simulink model "Copy_2_of_continuos_plant"  (R2016b)
settings: Solver=ode15s  StartTime=0.0  StopTime=200  FixedStep=0.01  RelTol=10^-1  AbsTol=10^-1
undefined symbols (not defined in the file or in its folder): deg, rad, s
libraries: simulink x6, aerolibconvert2 x2, dspsrcs4 x1, aerolib6dof2 x1
settings Model: Creator=Utente  LastModifiedBy=liana
settings SolverCC: SolverJacobianMethodControl=SparsePerturbation  SolverResetMethod=Robust
settings DataIOCC: SaveState=on
settings OptimizationCC: BlockReduction=off  DefaultParameterBehavior=Inlined  BufferReuse=off

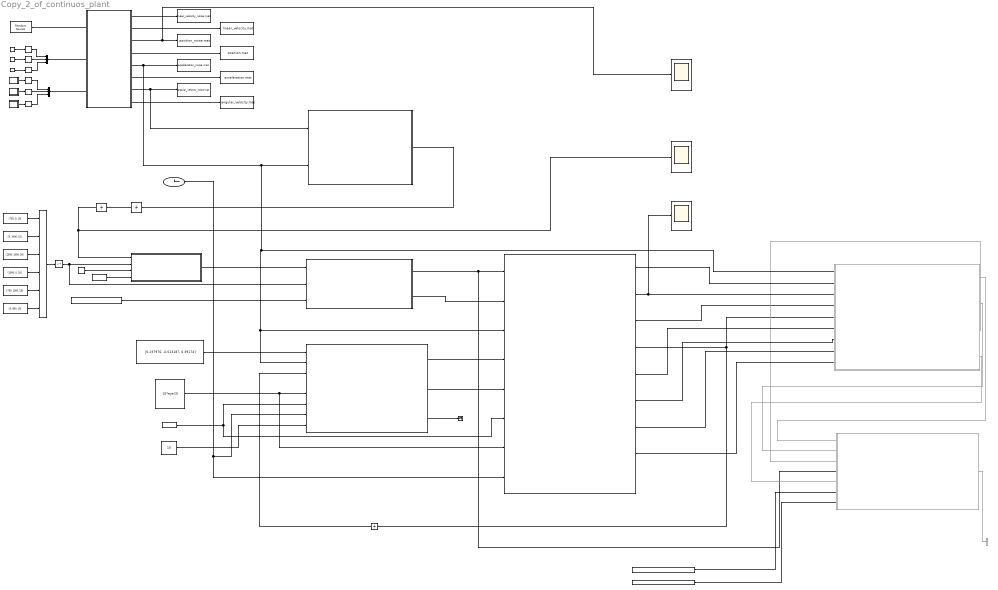
== system Copy_2_of_continuos_plant ==
  Attitude Observer : Subsystem
  Clock : Clock
      settings: Decimation=50
  Const : Constant
  Const1 : Constant  Value=0
  Const2 : Constant  Value=0
  Fx Slider : simulink/Math Operations/Slider Gain  low=-1  gain=1  high=1
  Fy Slider : simulink/Math Operations/Slider Gain  low=-1  gain=0  high=1
  Fz Slider : simulink/Math Operations/Slider Gain  low=-1  gain=0  high=1
  Integrator1 : Integrator  AbsoluteTolerance=10^-3
  Integrator2 : Integrator  AbsoluteTolerance=10^-3
  Kalman - Bucy Filter : Subsystem  Commented=on
  Kp : Constant  Value=10*eye(3)
  Local linearization1 : Subsystem  Commented=on
  Math Function : Math  Operator=transpose  SaturateOnIntegerOverflow=on
  Matrix Concatenate (transponders positions) : Concatenate  NumInputs=6  Mode=Multidimensional array  ConcatenateDimension=2
  Mechanisation subsystem : Subsystem
  Mux : Mux  Inputs=3
  Mux1 : Mux  Inputs=3
  Mxx Slider : simulink/Math Operations/Slider Gain  low=0  gain=0  high=1
  Myy Slider : simulink/Math Operations/Slider Gain  low=0  gain=0  high=1
  Mzz Slider : simulink/Math Operations/Slider Gain  low=-1  gain=1  high=3
  Nonlinear algebraic transform and solution : Subsystem
  Pitch moment : Subsystem  mask(timed input){t=[0 3 3 4 4 5 5  7.5 7.5 8.5 8.5 9.5 9.5 10], u=[0 0  1 1 -1 -1.005 0 0 -1 -1 1 1 0 0]*3.138/2}
      mask prompts: t "time values:"; u "input values"
      mask Display: plot(t,u)
  Position TMO : Scope
  "Position mechanisation " : Scope
  Position trajectory : Scope
  Q matrix : Constant  Value=diag([0, 0, 0, 10^-5, 10^-3, 10^-3, 10^-3, 10^-8, 10^-8, 10^-8])
  R matrix : Constant  Value=0.25*diag([1 1 1 1])
  Random Source : dspsrcs4/Random Source  SrcType=Gaussian  NormMethod=Ziggurat  CltLength=12  MinVal=0  MaxVal=1  MeanVal=[0.05 0.05 0.05]  VarVal=[5 5 5]  RepMode=Not repeatable  rawSeed=1  IsInherit=off  SampMode=Discrete  SampTime=1  SampFrame=1  DataType=Double  OutComplex=Real  OutputFrames=off
  Roll moment : Subsystem  mask(timed input){t=[0 1 1 2 2  10], u=[1 1 -1 -.998  0 0]*3.144/2}
      mask prompts: t "time values:"; u "input values"
      mask Display: plot(t,u)
  Terminator : Terminator
  Terminator2 : Terminator  Commented=on
  Translational Motion Observer : Subsystem
  Unit Delay : UnitDelay  SampleTime=-1
  Yaw moment : Subsystem  mask(timed input){t=[0 6 6 7 7 8 8 10], u=[0 0  -1 -1 1 1 0 0]*3.1/2}
      mask prompts: t "time values:"; u "input values"
      mask Display: plot(t,u)
  acceleration file : ToFile  Filename=acceleration_noise.mat  MatrixName=acc  SaveFormat=Timeseries
  acceleration file2 : ToFile  Filename=acceleration.mat  MatrixName=acc  SaveFormat=Timeseries
  angular velocity file : ToFile  Filename=angular_velocity_noise.mat  MatrixName=av  SaveFormat=Timeseries
  angular velocity file1 : ToFile  Filename=angular_velocity.mat  MatrixName=av  SaveFormat=Timeseries
  beta : Constant  Value=100
  epsilon : Constant  Value=[1 1 1 1 1 1]*0.1
  ki : Constant  Value=10
  magneto_values (Pisa) : Constant  Value=[0.237976, -0.013187, 0.39174]'
  p_n_1 : Constant  Value=[750, 0, 10]
  p_n_2 : Constant  Value=[0, 1000, 15]
  p_n_3 : Constant  Value=[1500, 1000, 30]
  p_n_4 : Constant  Value=[1500, 0, 20]
  p_n_5 : Constant  Value=[750, 1000, 25]
  p_n_6 : Constant  Value=[0, 600, 10]
  position file : ToFile  Filename=position_noise.mat  MatrixName=pos_noise  SaveFormat=Timeseries
  position file1 : ToFile  Filename=position.mat  MatrixName=pos  SaveFormat=Timeseries
  position_0_fixed_reference : Constant  Value=[4 5 5]
  pseudorange_measurement_model : MATLAB Function  TreatAsAtomicUnit=on
  sigma : Constant  Value=0.25
  trajectory : Subsystem
  velocity file : ToFile  Filename=linear_velocity_noise.mat  MatrixName=lv  SaveFormat=Timeseries
  velocity file1 : ToFile  Filename=linear_velocity.mat  MatrixName=lv  SaveFormat=Timeseries
  wires:
  Clock/1 -> Translational Motion Observer/8(t), Attitude Observer/7(t)
  Mechanisation subsystem/1(v_n_dot) -> Integrator1/1
  Nonlinear algebraic transform and solution/1(delta) -> Kalman - Bucy Filter/4(sensors measurements), Translational Motion Observer/1(delta)
  Translational Motion Observer/4(f_n_stim) -> Local linearization1/5(f_n_stim), Unit Delay/1
  Attitude Observer/1(J) -> Translational Motion Observer/4(J)
  Attitude Observer/2(R_nb_stim) -> Translational Motion Observer/5(R_nb_stim)
  Attitude Observer/3(b_stim) -> Terminator/1
  Kp/1 -> Translational Motion Observer/7(Kp), Attitude Observer/5(Kp)
  sigma/1 -> Attitude Observer/6(sigma), Translational Motion Observer/6(sigma)
  Translational Motion Observer/3(v_n_stim) -> Local linearization1/4(v_n_stim)
  Nonlinear algebraic transform and solution/2(C_dx) -> Translational Motion Observer/2(C_dx)
  Local linearization1/1(AL) -> Kalman - Bucy Filter/1(AL)
  Local linearization1/2(BL) -> Kalman - Bucy Filter/2(BL)
  Local linearization1/3(CL) -> Kalman - Bucy Filter/3(CL)
  pseudorange_measurement_model/1(y) -> Nonlinear algebraic transform and solution/1(y)
  Local linearization1/4(U) -> Kalman - Bucy Filter/5(U)
  beta/1 -> pseudorange_measurement_model/3(beta)
  epsilon/1 -> pseudorange_measurement_model/4(epsilon)
  Matrix Concatenate (transponders positions)/1 -> Math Function/1
  R matrix/1 -> Kalman - Bucy Filter/6(R)
  Q matrix/1 -> Kalman - Bucy Filter/7(Q)
  Kalman - Bucy Filter/1(Out1) -> Terminator2/1
  Translational Motion Observer/5(K) -> Local linearization1/6(K)
  Translational Motion Observer/6("C ") -> Local linearization1/7(C)
  Translational Motion Observer/7(" A") -> Local linearization1/8(A)
  Translational Motion Observer/8(B) -> Local linearization1/9(B)
  ki/1 -> Attitude Observer/8(Ki)
  Unit Delay/1 -> Attitude Observer/3(f_n_stim)
  Translational Motion Observer/1(beta_stim) -> Local linearization1/2(beta_stim)
  Translational Motion Observer/2(p_n_delta_stim) -> Position TMO/1, Local linearization1/3(p_n_stim)
  p_n_5/1 -> Matrix Concatenate (transponders positions)/5
  p_n_4/1 -> Matrix Concatenate (transponders positions)/4
  p_n_3/1 -> Matrix Concatenate (transponders positions)/3
  p_n_2/1 -> Matrix Concatenate (transponders positions)/2
  p_n_1/1 -> Matrix Concatenate (transponders positions)/1
  Math Function/1 -> pseudorange_measurement_model/2(p_n_i), Nonlinear algebraic transform and solution/2(p)
  trajectory/5(Acceleration_noise) -> Attitude Observer/2(f_b), Translational Motion Observer/3(f_b_imu), Local linearization1/1(f_b_imu), Mechanisation subsystem/2(f_b), acceleration file/1
  position_0_fixed_reference/1 -> Nonlinear algebraic transform and solution/3(p0)
  magneto_values (Pisa)/1 -> Attitude Observer/1(m_b_mag)
  Integrator1/1 -> Integrator2/1
  p_n_6/1 -> Matrix Concatenate (transponders positions)/6
  Integrator2/1 -> pseudorange_measurement_model/1(p_n), "Position mechanisation "/1
  Yaw moment/1(Out1) -> Mzz Slider/1
  Pitch moment/1(Out1) -> Myy Slider/1
  Roll moment/1(Out1) -> Mxx Slider/1
  Const2/1 -> Fz Slider/1
  Const1/1 -> Fy Slider/1
  Const/1 -> Fx Slider/1
  Mzz Slider/1 -> Mux1/3
  Myy Slider/1 -> Mux1/2
  Mxx Slider/1 -> Mux1/1
  Fy Slider/1 -> Mux/2
  Fz Slider/1 -> Mux/3
  Fx Slider/1 -> Mux/1
  Random Source/1 -> trajectory/1(Noise_output)
  Mux/1 -> trajectory/2(Force_xyz)
  Mux1/1 -> trajectory/3(M_xyz)
  trajectory/1(velocity_noise) -> velocity file/1
  trajectory/2(velocity) -> velocity file1/1
  trajectory/4(Position) -> position file1/1
  trajectory/6(Acceleration) -> acceleration file2/1
  trajectory/7(angular_velocity_noise) -> Mechanisation subsystem/1(w_ib), angular velocity file/1
  trajectory/8(angular_velocity) -> angular velocity file1/1
  trajectory/3(Position_noise) -> Position trajectory/1, position file/1

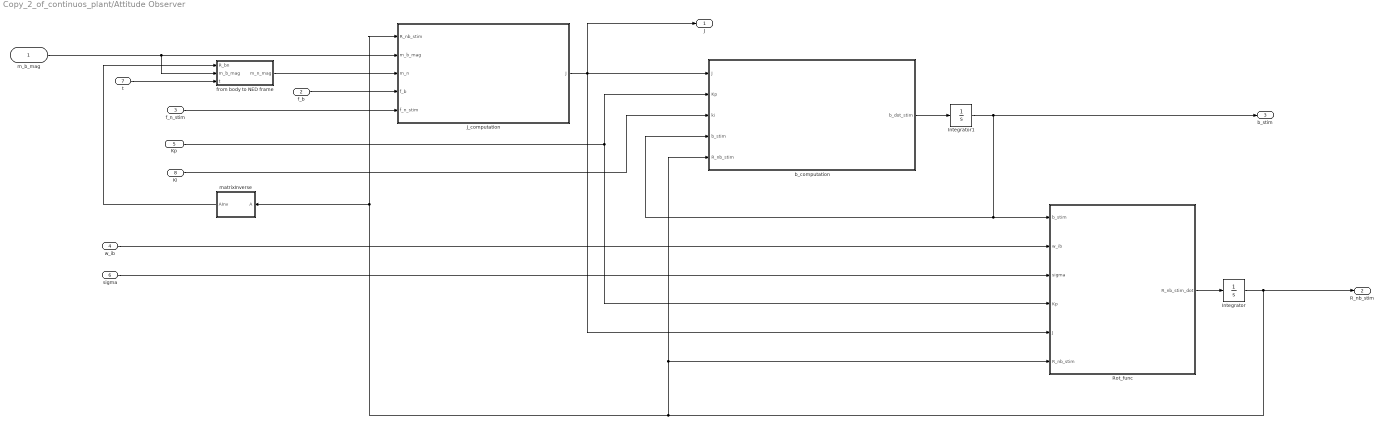
== system Copy_2_of_continuos_plant/Attitude Observer ==
  m_b_mag : Inport
  f_b : Inport  Port=2
  f_n_stim : Inport  Port=3
  w_ib : Inport  Port=4
  Kp : Inport  Port=5
  sigma : Inport  Port=6
  t : Inport  Port=7
  Ki : Inport  Port=8
  Integrator : Integrator  UpperSaturationLimit=1  LowerSaturationLimit=-1  AbsoluteTolerance=10^-1
  Integrator1 : Integrator  UpperSaturationLimit=100  LowerSaturationLimit=-100  AbsoluteTolerance=10^-2
  J_computation : Subsystem
  Rot_func : MATLAB Function  TreatAsAtomicUnit=on
  b_computation : MATLAB Function  TreatAsAtomicUnit=on
  from body to NED frame : MATLAB Function  TreatAsAtomicUnit=on
  matrixInverse : MATLAB Function  TreatAsAtomicUnit=on
  J : Outport
  R_nb_stim : Outport  Port=2
  b_stim : Outport  Port=3
  wires:
  m_b_mag/1 -> from body to NED frame/2(m_b_mag), J_computation/2(m_b_mag)
  from body to NED frame/1(m_n_mag) -> J_computation/3(m_n)
  f_b/1 -> J_computation/4(f_b)
  J_computation/1(J) -> J/1, Rot_func/5(J), b_computation/1(J)
  Kp/1 -> Rot_func/4(Kp), b_computation/2(Kp)
  Ki/1 -> b_computation/3(ki)
  sigma/1 -> Rot_func/3(sigma)
  w_ib/1 -> Rot_func/2(w_ib)
  t/1 -> from body to NED frame/3(t)
  Integrator1/1 -> Rot_func/1(b_stim), b_computation/4(b_stim), b_stim/1
  Integrator/1 -> Rot_func/6(R_nb_stim), b_computation/5(R_nb_stim), matrixInverse/1(A), J_computation/1(R_nb_stim), R_nb_stim/1
  b_computation/1(b_dot_stim) -> Integrator1/1
  Rot_func/1(R_nb_stim_dot) -> Integrator/1
  matrixInverse/1(AInv) -> from body to NED frame/1(R_bn)
  f_n_stim/1 -> J_computation/5(f_n_stim)

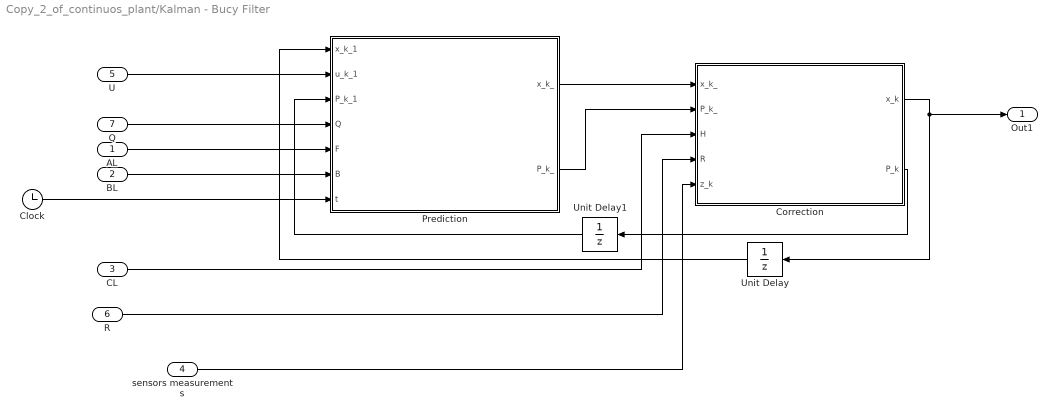
== system Copy_2_of_continuos_plant/Kalman - Bucy Filter ==
  AL : Inport
  BL : Inport  Port=2
  CL : Inport  Port=3
  sensors measurements : Inport  Port=4
  U : Inport  Port=5
  R : Inport  Port=6
  Q : Inport  Port=7
  Clock : Clock
  Correction : MATLAB Function  TreatAsAtomicUnit=on
  Prediction : MATLAB Function  TreatAsAtomicUnit=on
  Unit Delay : UnitDelay  SampleTime=-1
  Unit Delay1 : UnitDelay  SampleTime=-1
  Out1 : Outport
  wires:
  Prediction/2(P_k_) -> Correction/2(P_k_)
  Prediction/1(x_k_) -> Correction/1(x_k_)
  Correction/2(P_k) -> Unit Delay1/1
  Correction/1(x_k) -> Unit Delay/1, Out1/1
  AL/1 -> Prediction/5(F)
  CL/1 -> Correction/3(H)
  Clock/1 -> Prediction/7(t)
  Q/1 -> Prediction/4(Q)
  sensors measurements/1 -> Correction/5(z_k)
  BL/1 -> Prediction/6(B)
  U/1 -> Prediction/2(u_k_1)
  R/1 -> Correction/4(R)
  Unit Delay/1 -> Prediction/1(x_k_1)
  Unit Delay1/1 -> Prediction/3(P_k_1)

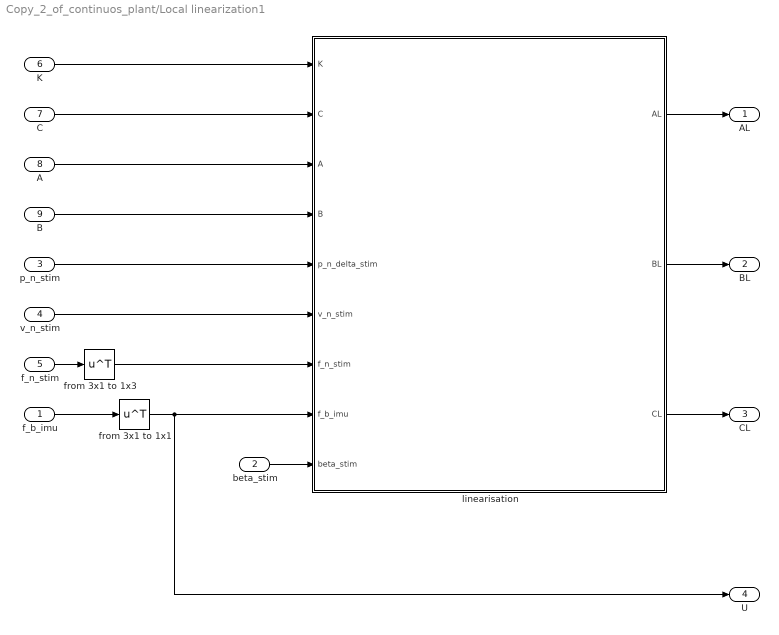
== system Copy_2_of_continuos_plant/Local linearization1 ==
  f_b_imu : Inport
  beta_stim : Inport  Port=2
  p_n_stim : Inport  Port=3
  v_n_stim : Inport  Port=4
  f_n_stim : Inport  Port=5
  K : Inport  Port=6
  C : Inport  Port=7
  A : Inport  Port=8
  B : Inport  Port=9
  from 3x1 to 1x1 : Math  Operator=transpose  SaturateOnIntegerOverflow=on
  from 3x1 to 1x3 : Math  Operator=transpose  SaturateOnIntegerOverflow=on
  linearisation : MATLAB Function  TreatAsAtomicUnit=on
  AL : Outport
  BL : Outport  Port=2
  CL : Outport  Port=3
  U : Outport  Port=4
  wires:
  linearisation/1(AL) -> AL/1
  linearisation/2(BL) -> BL/1
  linearisation/3(CL) -> CL/1
  K/1 -> linearisation/1(K)
  C/1 -> linearisation/2(C)
  A/1 -> linearisation/3(A)
  B/1 -> linearisation/4(B)
  p_n_stim/1 -> linearisation/5(p_n_delta_stim)
  beta_stim/1 -> linearisation/9(beta_stim)
  f_n_stim/1 -> from 3x1 to 1x3/1
  v_n_stim/1 -> linearisation/6(v_n_stim)
  f_b_imu/1 -> from 3x1 to 1x1/1
  from 3x1 to 1x3/1 -> linearisation/7(f_n_stim)
  from 3x1 to 1x1/1 -> U/1, linearisation/8(f_b_imu)

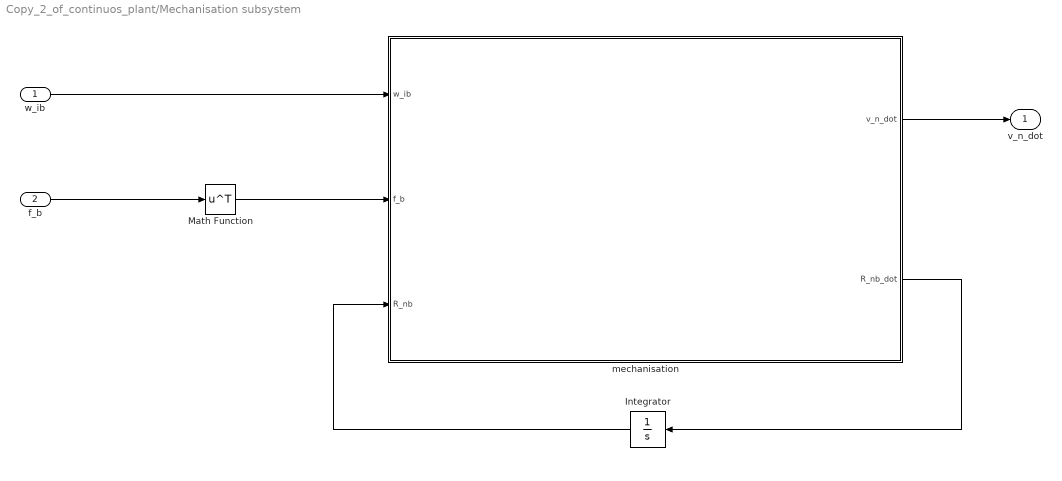
== system Copy_2_of_continuos_plant/Mechanisation subsystem ==
  w_ib : Inport
  f_b : Inport  Port=2
  Integrator : Integrator  AbsoluteTolerance=10^-3
  Math Function : Math  Operator=transpose  SaturateOnIntegerOverflow=on
  mechanisation : MATLAB Function  TreatAsAtomicUnit=on
  v_n_dot : Outport
  wires:
  w_ib/1 -> mechanisation/1(w_ib)
  f_b/1 -> Math Function/1
  mechanisation/1(v_n_dot) -> v_n_dot/1
  mechanisation/2(R_nb_dot) -> Integrator/1
  Integrator/1 -> mechanisation/3(R_nb)
  Math Function/1 -> mechanisation/2(f_b)

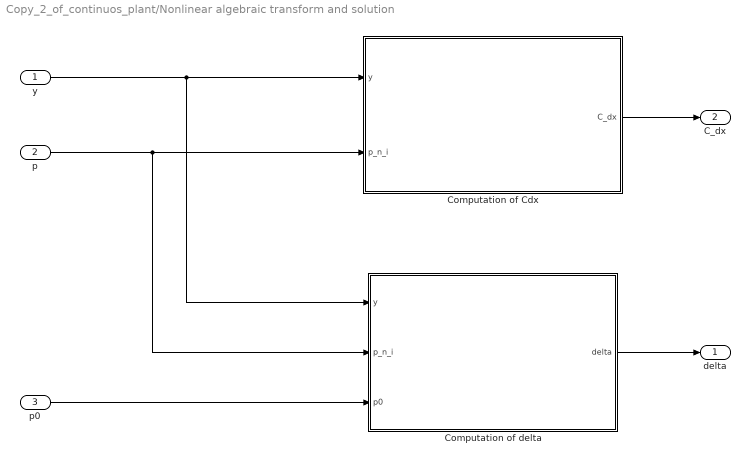
== system Copy_2_of_continuos_plant/Nonlinear algebraic transform and solution ==
  y : Inport
  p : Inport  Port=2
  p0 : Inport  Port=3
  Computation of Cdx : MATLAB Function  TreatAsAtomicUnit=on
  Computation of delta : MATLAB Function  TreatAsAtomicUnit=on
  delta : Outport
  C_dx : Outport  Port=2
  wires:
  y/1 -> Computation of delta/1(y), Computation of Cdx/1(y)
  p/1 -> Computation of delta/2(p_n_i), Computation of Cdx/2(p_n_i)
  p0/1 -> Computation of delta/3(p0)
  Computation of delta/1(delta) -> delta/1
  Computation of Cdx/1(C_dx) -> C_dx/1

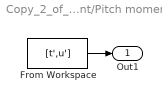
== system Copy_2_of_continuos_plant/Pitch moment ==
  From Workspace : FromWorkspace  VariableName=[t',u']  SampleTime=0
  Out1 : Outport
  wires:
  From Workspace/1 -> Out1/1

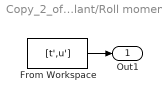
== system Copy_2_of_continuos_plant/Roll moment ==
  From Workspace : FromWorkspace  VariableName=[t',u']  SampleTime=0
  Out1 : Outport
  wires:
  From Workspace/1 -> Out1/1

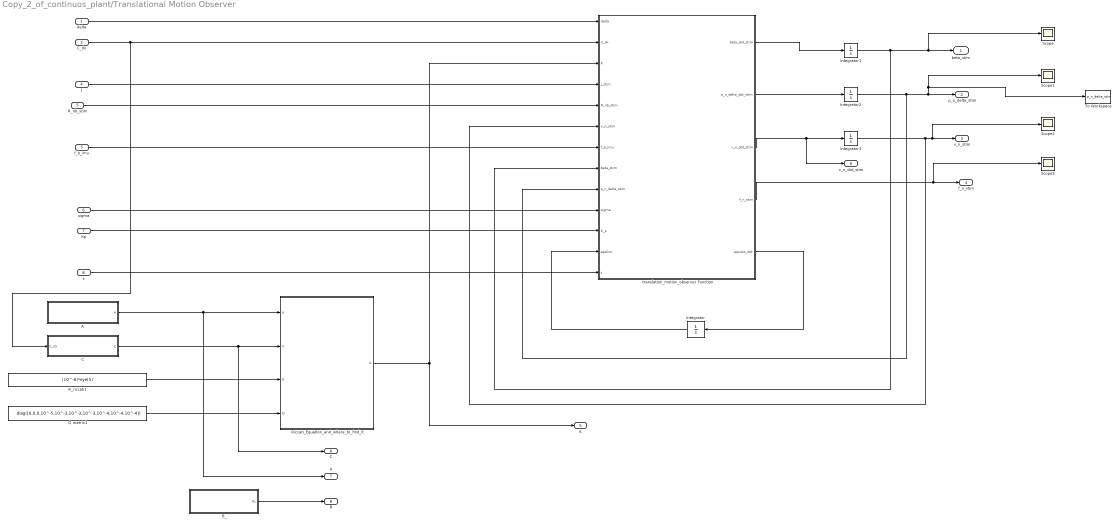
== system Copy_2_of_continuos_plant/Translational Motion Observer ==
  delta : Inport
  C_dx : Inport  Port=2
  f_b_imu : Inport  Port=3
  J : Inport  Port=4
  R_nb_stim : Inport  Port=5
  sigma : Inport  Port=6
  Kp : Inport  Port=7
  t : Inport  Port=8
  A : MATLAB Function  TreatAsAtomicUnit=on
  B_ : MATLAB Function  TreatAsAtomicUnit=on
  C : MATLAB Function  TreatAsAtomicUnit=on
  Integrator : Integrator  AbsoluteTolerance=10^-2
  Integrator1 : Integrator  AbsoluteTolerance=10^-3
  Integrator2 : Integrator  AbsoluteTolerance=10^-3
  Integrator3 : Integrator  AbsoluteTolerance=10^-3
  Q matrix1 : Constant  Value=diag([0,0,0,10^-5,10^-3,10^-3,10^-3,10^-4,10^-4,10^-4])
  R_riccati1 : Constant  Value=(10^-8)*eye(5)
  Riccati_Equation_and_where_to_find_it : Subsystem
  Scope{,1..3} (4 alike) : Scope
  To Workspace : ToWorkspace  VariableName=p_n_delta_stim  SaveFormat=Timeseries  SampleTime=-1
  translation_motion_observer Function : MATLAB Function  TreatAsAtomicUnit=on
  beta_stim : Outport
  p_n_delta_stim : Outport  Port=2
  v_n_stim : Outport  Port=3
  f_n_stim : Outport  Port=4
  K : Outport  Port=5
  "C " : Outport  Port=6
  " A" : Outport  Port=7
  B : Outport  Port=8
  v_n_dot_stim : Outport  Port=9
  wires:
  translation_motion_observer Function/4(f_n_stim) -> Scope3/1, f_n_stim/1
  translation_motion_observer Function/3(v_n_dot_stim) -> v_n_dot_stim/1, Integrator3/1
  translation_motion_observer Function/2(p_n_delta_dot_stim) -> Integrator2/1
  C_dx/1 -> C/1(C_dx), translation_motion_observer Function/2(C_dx)
  J/1 -> translation_motion_observer Function/4(J_stim)
  R_nb_stim/1 -> translation_motion_observer Function/5(R_nb_stim)
  delta/1 -> translation_motion_observer Function/1(delta)
  f_b_imu/1 -> translation_motion_observer Function/7(f_b_imu)
  sigma/1 -> translation_motion_observer Function/10(sigma)
  Kp/1 -> translation_motion_observer Function/11(K_p)
  A/1(A) -> " A"/1, Riccati_Equation_and_where_to_find_it/1("A ")
  C/1(C) -> "C "/1, Riccati_Equation_and_where_to_find_it/2(C)
  B_/1(B_) -> B/1
  t/1 -> translation_motion_observer Function/13(t)
  Integrator3/1 -> translation_motion_observer Function/6(v_n_stim), Scope2/1, v_n_stim/1
  translation_motion_observer Function/1(beta_dot_stim) -> Integrator1/1
  Integrator/1 -> translation_motion_observer Function/12(epsilon)
  Integrator1/1 -> Scope/1, beta_stim/1, translation_motion_observer Function/8(beta_stim)
  translation_motion_observer Function/5(epsilon_dot) -> Integrator/1
  Integrator2/1 -> translation_motion_observer Function/9(p_n_delta_stim), To Workspace/1, Scope1/1, p_n_delta_stim/1
  Riccati_Equation_and_where_to_find_it/1(K) -> translation_motion_observer Function/3(K), K/1
  Q matrix1/1 -> Riccati_Equation_and_where_to_find_it/4("Q ")
  R_riccati1/1 -> Riccati_Equation_and_where_to_find_it/3("R ")

== system Copy_2_of_continuos_plant/Yaw moment ==
  From Workspace : FromWorkspace  VariableName=[t',u']  SampleTime=0
  Out1 : Outport
  wires:
  From Workspace/1 -> Out1/1

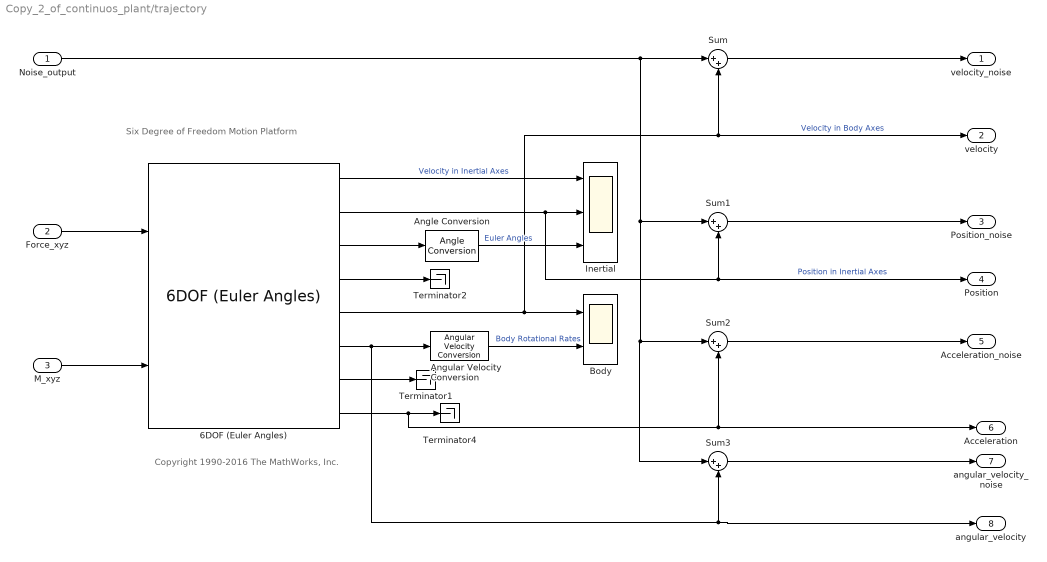
== system Copy_2_of_continuos_plant/trajectory ==
  note: Six Degree of Freedom Motion Platform
  note: Copyright 1990-2016 The MathWorks, Inc.
  Noise_output : Inport
  Force_xyz : Inport  Port=2
  M_xyz : Inport  Port=3
  6DOF (Euler Angles) : aerolib6dof2/6DOF (Euler Angles)  units=Metric (MKS)  mtype=Fixed  rep=Euler Angles  xme_0=[0 0 0]  Vm_0=[0 0 0]  eul_0=[0 0 0]  pm_0=[0 0 0]  mass_0=1.0  mass_e=0.5  mass_f=2.0  inertia=eye(3)  inertia_e=eye(3)  inertia_f=2*eye(3)  k_quat=1.0  vre_flag=on
  Angle Conversion : aerolibconvert2/Angle Conversion  IU=rad  OU=deg
  Angular Velocity Conversion : aerolibconvert2/Angular Velocity Conversion  IU=rad/s  OU=deg/s
  Body : Scope  NumInputPorts=2
  Inertial : Scope  NumInputPorts=3
  Sum{,1..3} (4 alike) : Sum  Inputs=|++
  Terminator1 : Terminator
  Terminator2 : Terminator
  Terminator4 : Terminator
  velocity_noise : Outport
  velocity : Outport  Port=2
  Position_noise : Outport  Port=3
  Position : Outport  Port=4
  Acceleration_noise : Outport  Port=5
  Acceleration : Outport  Port=6
  angular_velocity_noise : Outport  Port=7
  angular_velocity : Outport  Port=8
  wires:
  6DOF (Euler Angles)/8 -> Sum2/2, Acceleration/1, Terminator4/1
  Sum/1 -> velocity_noise/1
  Noise_output/1 -> Sum3/1, Sum2/1, Sum1/1, Sum/1
  6DOF (Euler Angles)/3 -> Angle Conversion/1
  6DOF (Euler Angles)/5 -> Sum/2, velocity/1, Body/1  "Velocity in Body Axes"
  Sum3/1 -> angular_velocity_noise/1
  Force_xyz/1 -> 6DOF (Euler Angles)/1
  Sum1/1 -> Position_noise/1
  6DOF (Euler Angles)/6 -> angular_velocity/1, Sum3/2, Angular Velocity Conversion/1
  Angular Velocity Conversion/1 -> Body/2  "Body Rotational Rates"
  6DOF (Euler Angles)/7 -> Terminator1/1
  6DOF (Euler Angles)/2 -> Position/1, Sum1/2, Inertial/2  "Position in Inertial Axes"
  6DOF (Euler Angles)/4 -> Terminator2/1
  Sum2/1 -> Acceleration_noise/1
  Angle Conversion/1 -> Inertial/3  "Euler Angles"
  6DOF (Euler Angles)/1 -> Inertial/1  "Velocity in Inertial Axes"
  M_xyz/1 -> 6DOF (Euler Angles)/2

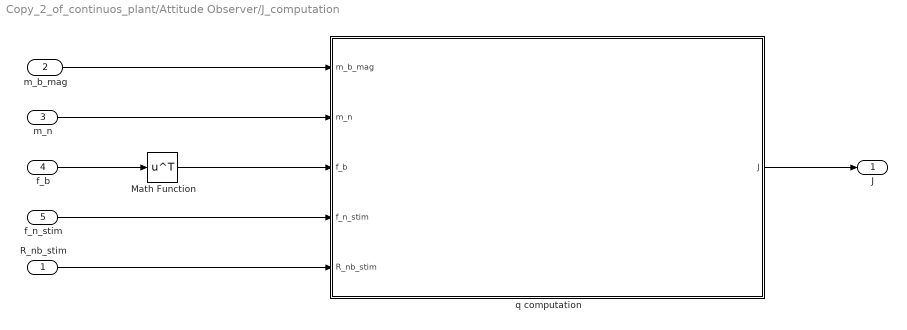
== system Copy_2_of_continuos_plant/Attitude Observer/J_computation ==
  R_nb_stim : Inport
  m_b_mag : Inport  Port=2
  m_n : Inport  Port=3
  f_b : Inport  Port=4
  f_n_stim : Inport  Port=5
  Math Function : Math  Operator=transpose  SaturateOnIntegerOverflow=on
  q computation : MATLAB Function  TreatAsAtomicUnit=on
  J : Outport
  wires:
  m_n/1 -> q computation/2(m_n)
  f_n_stim/1 -> q computation/4(f_n_stim)
  m_b_mag/1 -> q computation/1(m_b_mag)
  f_b/1 -> Math Function/1
  q computation/1(J) -> J/1
  R_nb_stim/1 -> q computation/5(R_nb_stim)
  Math Function/1 -> q computation/3(f_b)

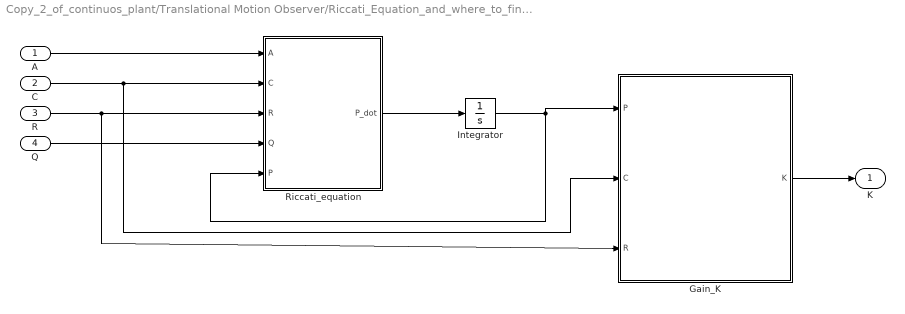
== system Copy_2_of_continuos_plant/Translational Motion Observer/Riccati_Equation_and_where_to_find_it ==
  "A " : Inport
  C : Inport  Port=2
  "R " : Inport  Port=3
  "Q " : Inport  Port=4
  Gain_K : MATLAB Function  TreatAsAtomicUnit=on
  Integrator : Integrator
  Riccati_equation : MATLAB Function  TreatAsAtomicUnit=on
  K : Outport
  wires:
  Gain_K/1(K) -> K/1
  Riccati_equation/1(P_dot) -> Integrator/1
  Integrator/1 -> Riccati_equation/5(P), Gain_K/1(P)
  "Q "/1 -> Riccati_equation/4(Q)
  "R "/1 -> Gain_K/3(R), Riccati_equation/3(R)
  C/1 -> Gain_K/2(C), Riccati_equation/2(C)
  "A "/1 -> Riccati_equation/1(A)

== matlab function Copy_2_of_continuos_plant/Translational Motion Observer/Riccati_Equation_and_where_to_find_it/Riccati_equation ==
  data: A input; C input; P_dot output; R input; Q input; P input
function P_dot = fcn(A,C,R,Q,P)

P_dot = P*A+A'*P-P*C'*inv(R)*C*P+Q;

== matlab function Copy_2_of_continuos_plant/Attitude Observer/J_computation/q computation ==
  data: m_b_mag input; m_n input; f_b input; f_n_stim input size=3; J output; R_nb_stim input size=[3,3]
function J  = qEfunc(m_b_mag, m_n, f_b, f_n_stim, R_nb_stim)

g_n = [0 0 9.81]';

q1_b = m_b_mag/norm(m_b_mag,2);
q2_b = f_b/norm(g_n,2);

q1_n = m_n/norm(m_n,2);
q2_n = f_n_stim/norm(g_n,2);


E_b = [q1_b, skew(q1_b)*q2_b, (skew(q1_b)*skew(q1_b))*q2_b];
E_n = [q1_n, skew(q1_n)*q2_n, (skew(q1_n)*skew(q1_n))*q2_n];

J = (E_n - R_nb_stim * E_b) * (E_b');

end

== matlab function Copy_2_of_continuos_plant/Kalman - Bucy Filter/Prediction ==
  data: x_k_1 input size=[10, 1]; x_k_ output; u_k_1 input; P_k_1 input size=[10,10]; Q input; F input; B input; P_k_ output; t input
function [x_k_, P_k_] = prediction(x_k_1, u_k_1, P_k_1, Q, F,B, t)

    % initial value of x_k_1
    if t == 0
        x_k_1 = zeros(10,1);
    end

    x_k_ = F * x_k_1 + B * u_k_1';
    
    P_k_ = F * P_k_1 * F' + Q;
    

end

== matlab function Copy_2_of_continuos_plant/Translational Motion Observer/Riccati_Equation_and_where_to_find_it/Gain_K ==
  data: P input; K output; C input; R input
function K = fcn(P,C,R)

K = P*C'*inv(R);

== matlab function Copy_2_of_continuos_plant/Mechanisation subsystem/mechanisation ==
  data: w_ib input; f_b input; v_n_dot output; R_nb_dot output; R_nb input
function [v_n_dot, R_nb_dot] = mechanisation(w_ib, f_b, R_nb)

g_n = [0 0 9.81]';
% 
% if t == 0
%     v_n_dot = zeros(3,1);
%     R_nb_dot = eye(3);
%     R_nb = eye(3);
% end

Skew = skew(w_ib);

v_n_dot = R_nb * f_b + g_n;

R_nb_dot = R_nb * Skew;

== matlab function Copy_2_of_continuos_plant/Attitude Observer/b_computation ==
  data: J input; b_dot_stim output size=3; Kp input; ki input; b_stim input; R_nb_stim input
function b_dot_stim  = b_dot_stim_func(J, Kp, ki, b_stim, R_nb_stim)

SAT = sat(R_nb_stim);
PA = pa( SAT' * Kp * J);
VEX = vexfunc(PA);
b_dot_stim = Proj(b_stim , -ki * VEX);
% b_dot_stim = Proj(-ki * VEX, 0.5);

end

== matlab function Copy_2_of_continuos_plant/Translational Motion Observer/translation_motion_observer Function ==
  data: delta input; C_dx input; K input; beta_dot_stim output; J_stim input; R_nb_stim input; p_n_delta_dot_stim output; v_n_dot_stim output; f_n_stim output size=[3,1]; v_n_stim input size=3; f_b_imu input size=3; beta_stim input; p_n_delta_stim input size=3; sigma input; K_p input; epsilon_dot output; epsilon input size=3; t input
function [beta_dot_stim,p_n_delta_dot_stim,v_n_dot_stim,f_n_stim,epsilon_dot] =  TMO_func(delta,C_dx,K,J_stim,R_nb_stim, v_n_stim,f_b_imu, beta_stim, p_n_delta_stim,sigma,K_p,epsilon,t)

 K_pp = K(1:3,:); 
 K_beta_p = K(4,:);
 K_v_p = K(5:7,:);
 K_eps_p = K(8:10,:);
 %obtained by Riccati equation..


% remember to insert a clock to define dimensions of all variables
g_n = [0 0 9.81]';

if(t == 0)   
    delta_stim = zeros(3, 1);
    delta_diff = zeros(3, 1);
    v_n_stim = zeros(3, 1);
    beta_stim = 0;
    epsilon = zeros(3,1);
    p_n_delta_stim = zeros(3, 1);
end

x_stim = [p_n_delta_stim; beta_stim];


p_n_delta_dot_stim = v_n_stim + K_pp * (delta - 2*C_dx*x_stim); % eq 14
beta_dot_stim = K_beta_p * (delta - 2*C_dx*x_stim);             % eq 15
f_n_stim = R_nb_stim * f_b_imu + epsilon ;         % eq 18
v_n_dot_stim  = f_n_stim + g_n + K_v_p*(delta - 2*C_dx*x_stim);    % eq 16
epsilon_dot   = -sigma * K_p * J_stim *f_b_imu + K_eps_p * (delta - 2*C_dx * x_stim); % eq 17

end

== matlab function Copy_2_of_continuos_plant/Nonlinear algebraic transform and solution/Computation of Cdx ==
  data: y input; p_n_i input; C_dx output size=[5,4]
function C_dx  = C_dx_func(y,p_n_i)

    % y vector 
    % p matrix has row vectors
    %            (x,y,z) cols 
    %            m-rows are transponders number
    % all variables are in navigation frame oh yeah! baby ;)
    
    [row,col] = size(p_n_i);
    [row_,col_] = size(y);
    
    % m-measure vector
    p_m = p_n_i(row,:); % measure of m-th transponder
    y_m = y(row_);  % m-th pseudorange measure

    m = row; % m is transpoders number
    
    p_ = zeros(m-1,3); %row vector, 3 stands for x,y,z
    y_ = zeros(m-1,1);
    
    for i = 1 : 1 : m-1
    
        p_(i,:) = p_m - p_n_i(i,:);
        y_(i) = y(i) - y_m;
        
    end
    
    C_dx = [p_, y_];

end

== matlab function Copy_2_of_continuos_plant/Nonlinear algebraic transform and solution/Computation of delta ==
  data: y input; delta output size=5; p_n_i input; p0 input
function delta  = delta_func(y, p_n_i, p0)

    % y vector 
    % p matrix has row vectors
    %            (x,y,z) cols 
    %            m-rows are the numbers of the transponders
    % all variables are in navigation frame oh yeah! baby ;)
    % z is a col vector of scalars
    % we must choose p0 (a block)
    
    [row,col] = size(p_n_i);
    %[row_,col_] = size(y);
    
    p_los = zeros(row,col);
    z = zeros(row,1);   % dim = m x 1
    
    %defining los vector
    for i = 1:1:row
       p_los(i,:) = p_n_i(i,:) - p0';       % dim = m x 3
    end
    
    for i = 1:1:row
        p_los_norm = norm(p_los(i,:))^2;
        z(i)= (y(i)^2) - p_los_norm; % dim = m x 1
    end
    
    delta = zeros(row-1,1); %dim = (m-1) x 1
    z_m = z(row,1);
    
    for i=1:1:(row-1)
        delta(i,1) = z(i,1) - z_m;
    end

end

== matlab function Copy_2_of_continuos_plant/Attitude Observer/Rot_func ==
  data: b_stim input; R_nb_stim_dot output; w_ib input; sigma input; Kp input; J input; R_nb_stim input
function R_nb_stim_dot = rot_func(b_stim,w_ib,sigma,Kp,J,R_nb_stim) 

Skew = skew(w_ib - b_stim);

R_nb_stim_dot = R_nb_stim * Skew + sigma * Kp * J;

== matlab function Copy_2_of_continuos_plant/Kalman - Bucy Filter/Correction ==
  data: x_k_ input; P_k_ input size=[10,10]; H input; R input; z_k input; x_k output; P_k output
function [x_k, P_k] = correction(x_k_ ,P_k_, H, R, z_k)

    n = size(P_k_);


    K_k = P_k_ * H' * pinv(H * P_k_ * H' + R);
    
    x_k = x_k_ + K_k * (z_k - H * x_k_);
    
    P_k = (eye(n) - K_k * H)*P_k_;

end

== matlab function Copy_2_of_continuos_plant/Translational Motion Observer/A ==
  data: A output
function A = A()

 A = zeros(10);

 A(1:3,5:7) = eye(3);
 A(5:7,8:10) = eye(3);
 
end

== matlab function Copy_2_of_continuos_plant/Translational Motion Observer/C ==
  data: C output; C_dx input
function C = Cfunc(C_dx)

   row = size(C_dx,1); 

   C1 = zeros(row,6);

 C = [2*C_dx C1];
 
 
end

== matlab function Copy_2_of_continuos_plant/Translational Motion Observer/B_ ==
  data: B_ output
function B_ = B()

 B_ = zeros(10,3);

 B_(8:10,1:3) = eye(3);
end

== matlab function Copy_2_of_continuos_plant/pseudorange_measurement_model ==
  data: p_n input; y output size=[6,1]; p_n_i input; beta input; epsilon input
function y = pseudorange_mea_model(p_n, p_n_i, beta, epsilon)

  %  row-vector

  y = zeros(size(p_n_i,1),1);

  for i = 1:1:size(p_n_i,1)

      rho = norm(p_n - (p_n_i(i,:))');  % eq. 7
      
      y(i) = rho + beta + epsilon(i); % eq. 8 

  end
      
end

== matlab function Copy_2_of_continuos_plant/Local linearization1/linearisation ==
  data: K input size=[10,4]; AL output size=[10,10]; BL output size=[10,3]; CL output size=[4,10]; C input size=[4,10]; A input size=[10,10]; B input size=[10,3]; p_n_delta_stim input size=[1,3]; v_n_stim input size=[1,3]; f_n_stim input size=[1,3]; f_b_imu input size=[1,3]; beta_stim input size=1
function [AL, BL, CL] = linearisation(K,C,A,B, p_n_delta_stim, v_n_stim, f_n_stim, f_b_imu, beta_stim)

 % building state vector
 % xsi = [p_n_stim ; beta_stim; v_n_stim; f_n_tim];
%   xsi = zeros(10,1);
%   xsi(1:3,1) = p_n_delta_stim;
%   xsi(4,1) = beta_stim;
%   xsi(5:7,1) = v_n_stim;
%   xsi(8:10,1) = f_n_stim;
 % coder.extrinsic('ss');
 % sys = ss(A-K*C,B,C,0);
% % getting work point
%coder.extrinsic('trim');
%[X,U,Y,DX] = trim('sys', xsi);

% computing linearisation model
%coder.extrinsic('linmod');
%[AL, BL, CL, DL] = linmod('sys',X,U);

  
AL = zeros(10,10);
BL = zeros(10,3);
CL = zeros(size(C,1), 10);


coder.extrinsic('LinearizationFun');

[Al,Bl,Cl] = LinearizationFun(K,C,A,B);

p_n0 = p_n_delta_stim(1, 1);
p_n1 = p_n_delta_stim (1,2);
p_n2 = p_n_delta_stim(1,3);

v_n0 = v_n_stim(1, 1);
v_n1 = v_n_stim(1,2);
v_n2 = v_n_stim(1,3);

f_n0 = f_n_stim(1,1);
f_n1 = f_n_stim(1,2);
f_n2 = f_n_stim(1,3);

f_b0 = f_b_imu(1,1);
f_b1 = f_b_imu(1,2);
f_b2 = f_b_imu(1,3);


coder.extrinsic('eval');

AL_ = eval(Al);
BL_ = eval(Bl);
CL_ = eval(Cl);

% AL_ = feval('Al', p_n0, p_n1, p_n2,v_n0, v_n1, v_n2, f_n0, f_n1, f_n2, beta_stim);
% BL_ = feval('Bl', f_b0, f_b1, f_b2);
% CL_ = feval('Cl', p_n0, p_n1, p_n2,v_n0, v_n1, v_n2, f_n0, f_n1, f_n2, beta_stim);
% 

AL = AL_;
BL = BL_;
CL = CL_;


end

== matlab function Copy_2_of_continuos_plant/Attitude Observer/from body to NED frame ==
  data: R_bn input; m_n_mag output; m_b_mag input; t input
function m_n_mag = b2n(R_bn, m_b_mag, t)

% m_n_mag and m_b_mag are 3x1

if t==0
    R_bn = eye(3);
end

m_n_mag = R_bn * m_b_mag;

== matlab function Copy_2_of_continuos_plant/Attitude Observer/matrixInverse ==
  data: A input; AInv output
function AInv  = matrixInverse(A)

% inverse by singular value decomposition


[n,m] = size(A);

% U = zeros(n,n);
% V = zeros(n,n);
% S = zeros(n,n);

[U,S,V] = svd(A);

pos = 0;

% maximun admissible condition number
csi = 10^3;

for i=n:-1:1
    if( S(1,1)/S(i,i) > csi)
        S(i,i) = 0;
        pos = i; % keeps the last eliminated singular value
    end
end

tempS = S(1:pos-1,1:pos-1); %take the non-zero set
tempS = inv(tempS);
S(1:pos-1,1:pos-1) = tempS(1:pos-1,1:pos-1); % now S is the inverse matrix
AInv = V * S * U';

end
